simulink model "scenarioCloseLoop_supervisoryACC"  (R2019b)
settings: Solver=FixedStepAuto  StartTime=0.0  StopTime=30  FixedStep=0.01  RelTol=1e-3
PreLoadFcn:
  | Ts1 = 0.01;
  | Ts2 = 0.1;
InitFcn:
  | initACCParams_pid;
  | Ts1 = 0.01;
  | Ts2 = 0.1;
model workspace (MAT data in the model file):
  firstWarning = 1
  originalScenarioChecksum = '3C3E23DDE530CB8BEC76DD6DBB66960A'
undefined symbols (not defined in the file): APP_gain, BPP_gain, m, sigbuilder_block, steer_gain
libraries: drivingscenarioandsensors x2, autolibshared x1, vehdynlibviscommon x1
settings Model: SILPILSystemUnderTest=refmodels  EnablePacing=on  Creator=sseshadr  LastModifiedBy=cdsouza
settings OptimizationCC: DefaultParameterBehavior=Inlined  EnhancedBackFolding=on  PassReuseOutputArgsAs=Individual arguments  ZeroExternalMemoryAtStartup=off  ZeroInternalMemoryAtStartup=off  OptimizeBlockOrder=speed  DifferentSizesBufferReuse=on  OptimizationCustomize=off  EfficientTunableParamExpr=on
settings DebuggingCC: ParameterTunabilityLossMsg=error
settings SFSimCC: MATLABDynamicMemAlloc=off
settings RTWCC: SystemTargetFile=ert.tlc  TemplateMakefile=ert_default_tmf  GenerateReport=on  IncludeHyperlinkInReport=on  LaunchReport=on  PortableWordSizes=on  CreateSILPILBlock=SIL  CodeExecutionProfiling=on  CodeProfilingInstrumentation=coarse  GenerateTraceInfo=on  GenerateTraceReport=on  GenerateTraceReportSl=on  GenerateTraceReportSf=on  GenerateTraceReportEml=on
settings CodeAppCC: ForceParamTrailComments=on  IgnoreCustomStorageClasses=off  OperatorAnnotations=on  SimulinkDataObjDesc=on  SFDataObjDesc=on  InsertBlockDesc=on
settings ERTTargetCC: TargetLangStandard=C99 (ISO)  GenerateSampleERTMain=on  InlinedParameterPlacement=NonHierarchical  ERTCustomFileTemplate=example_file_process.tlc

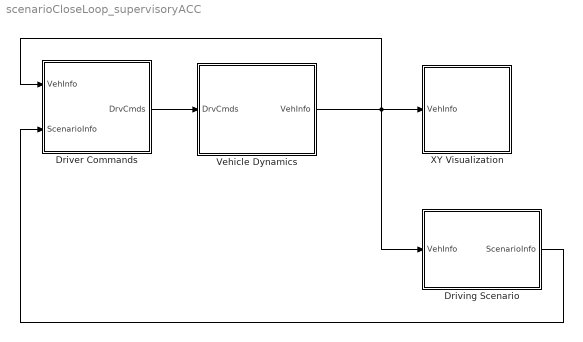
== system scenarioCloseLoop_supervisoryACC ==
  Driver Commands : Subsystem
  Driving Scenario : Subsystem
  Vehicle Dynamics : Subsystem
  XY Visualization : Subsystem
  wires:
  Driving Scenario/1(ScenarioInfo) -> Driver Commands/2(ScenarioInfo)
  Vehicle Dynamics/1(VehInfo) -> Driving Scenario/1(VehInfo), Driver Commands/1(VehInfo), XY Visualization/1(VehInfo)
  Driver Commands/1(DrvCmds) -> Vehicle Dynamics/1(DrvCmds)

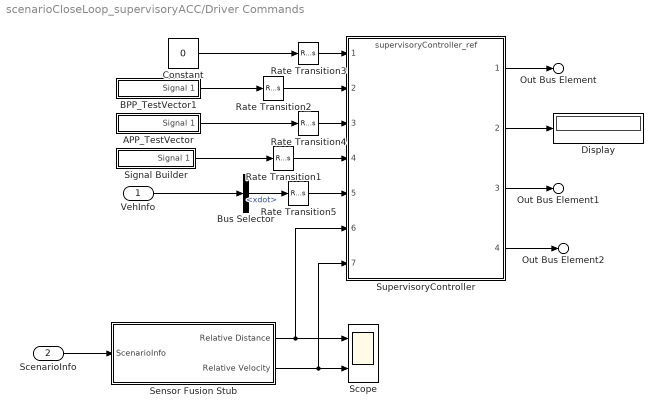
== system scenarioCloseLoop_supervisoryACC/Driver Commands ==
  VehInfo : Inport
  ScenarioInfo : Inport  Port=2
  APP_TestVector : Subsystem  Tag=STV Subsys  LoadFcn=sigbuilder_block('load');  StartFcn=sigbuilder_block('start');  StopFcn=sigbuilder_block('stop');  ClipboardFcn=sigbuilder_block('clipboard');  mask(Sigbuilder block){tuvar=[0:10]}
      mask help: Simulink:masks:SigbuilderBlock_MD
      mask init:
      | if ~strcmp(get_param(bdroot(gcbh),'SimulationStatus'),'stopped') tuvar = sigbuilder_block('maskInit'); end
      settings: CopyFcn=sigbuilder_block('copy');  DeleteFcn=sigbuilder_block('delete');  ModelCloseFcn=sigbuilder_block('modelClose');  PreSaveFcn=sigbuilder_block('preSave');  PauseFcn=sigbuilder_block('pause');  ContinueFcn=sigbuilder_block('continue');  NameChangeFcn=sigbuilder_block('namechange');  OpenFcn=sigbuilder_block('open',[609 515.25 550.5 237.75 ]);  CloseFcn=sigbuilder_block('close');
      mask Display: plot(0, 0, 100, 100,[2, 2, 32, 32, 2], [68, 8, 8, 68, 68],[32, 2], [38, 38], [32, 19, 2],[53, 60, 44], [32, 17, 17, 2],[16, 16, 31, 31]);txt = getActiveGroup(gcbh);text(2, 100, txt,'verticalAlignment', 'top');
  BPP_TestVector1 : Subsystem  Tag=STV Subsys  LoadFcn=sigbuilder_block('load');  StartFcn=sigbuilder_block('start');  StopFcn=sigbuilder_block('stop');  ClipboardFcn=sigbuilder_block('clipboard');  mask(Sigbuilder block){tuvar=[0:10]}
      mask help: Simulink:masks:SigbuilderBlock_MD
      mask init:
      | if ~strcmp(get_param(bdroot(gcbh),'SimulationStatus'),'stopped') tuvar = sigbuilder_block('maskInit'); end
      settings: CopyFcn=sigbuilder_block('copy');  DeleteFcn=sigbuilder_block('delete');  ModelCloseFcn=sigbuilder_block('modelClose');  PreSaveFcn=sigbuilder_block('preSave');  PauseFcn=sigbuilder_block('pause');  ContinueFcn=sigbuilder_block('continue');  NameChangeFcn=sigbuilder_block('namechange');  OpenFcn=sigbuilder_block('open',[325.5 304.5 550.5 278.25 ]);  CloseFcn=sigbuilder_block('close');
      mask Display: plot(0, 0, 100, 100,[2, 2, 32, 32, 2], [68, 8, 8, 68, 68],[32, 2], [38, 38], [32, 19, 2],[53, 60, 44], [32, 17, 17, 2],[16, 16, 31, 31]);txt = getActiveGroup(gcbh);text(2, 100, txt,'verticalAlignment', 'top');
  Bus Selector : BusSelector  OutputSignals=BdyFrm.Cg.Vel.xdot
  Constant : Constant  Value=0  SampleTime=0.01
  Display : Display
  Rate Transition{1..5} (5 alike) : RateTransition  OutPortSampleTime=0.01
  Scope : Scope  NumInputPorts=2
  Sensor Fusion Stub : Subsystem
  Signal Builder : Subsystem  Tag=STV Subsys  LoadFcn=sigbuilder_block('load');  StartFcn=sigbuilder_block('start');  StopFcn=sigbuilder_block('stop');  ClipboardFcn=sigbuilder_block('clipboard');  mask(Sigbuilder block){tuvar=[0:10]}
      mask help: Simulink:masks:SigbuilderBlock_MD
      mask init:
      | if ~strcmp(get_param(bdroot(gcbh),'SimulationStatus'),'stopped') tuvar = sigbuilder_block('maskInit'); end
      settings: CopyFcn=sigbuilder_block('copy');  DeleteFcn=sigbuilder_block('delete');  ModelCloseFcn=sigbuilder_block('modelClose');  PreSaveFcn=sigbuilder_block('preSave');  PauseFcn=sigbuilder_block('pause');  ContinueFcn=sigbuilder_block('continue');  NameChangeFcn=sigbuilder_block('namechange');  OpenFcn=sigbuilder_block('open',[401.25 280.5 550.5 278.25 ]);  CloseFcn=sigbuilder_block('close');
      mask Display: plot(0, 0, 100, 100,[2, 2, 32, 32, 2], [68, 8, 8, 68, 68],[32, 2], [38, 38], [32, 19, 2],[53, 60, 44], [32, 17, 17, 2],[16, 16, 31, 31]);txt = getActiveGroup(gcbh);text(2, 100, txt,'verticalAlignment', 'top');
  SupervisoryController : ModelReference  ModelNameDialog=supervisoryController_ref  SimulationMode=Normal  ModelReferenceVersion=1.30
  Out Bus Element : Outport  PortName=DrvCmds  Element=SteerCmd
  Out Bus Element1 : Outport  PortName=DrvCmds  Element=BPP Pedal
  Out Bus Element2 : Outport  PortName=DrvCmds  Element=APP Pedal
  wires:
  ScenarioInfo/1 -> Sensor Fusion Stub/1(ScenarioInfo)
  VehInfo/1 -> Bus Selector/1
  Sensor Fusion Stub/1(Relative Distance) -> SupervisoryController/6, Scope/1
  Sensor Fusion Stub/2(Relative Velocity) -> SupervisoryController/7, Scope/2
  Bus Selector/1 -> Rate Transition5/1  "<xdot>"
  SupervisoryController/1 -> Out Bus Element/1
  SupervisoryController/2 -> Display/1
  SupervisoryController/3 -> Out Bus Element1/1
  SupervisoryController/4 -> Out Bus Element2/1
  Rate Transition4/1 -> SupervisoryController/3
  Rate Transition2/1 -> SupervisoryController/2
  Rate Transition3/1 -> SupervisoryController/1
  Rate Transition5/1 -> SupervisoryController/5
  Signal Builder/1(Signal 1) -> Rate Transition1/1
  APP_TestVector/1(Signal 1) -> Rate Transition4/1
  Constant/1 -> Rate Transition3/1
  BPP_TestVector1/1(Signal 1) -> Rate Transition2/1
  Rate Transition1/1 -> SupervisoryController/4

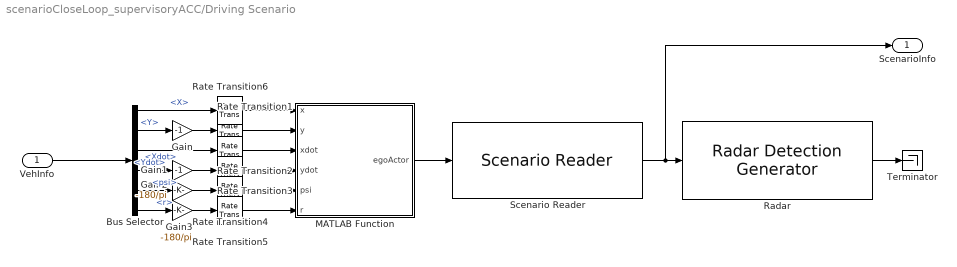
== system scenarioCloseLoop_supervisoryACC/Driving Scenario ==
  VehInfo : Inport
  Bus Selector : BusSelector  OutputSignals=InertFrm.Cg.Disp.X,InertFrm.Cg.Disp.Y,InertFrm.Cg.Vel.Xdot,InertFrm.Cg.Vel.Ydot,InertFrm.Cg.Ang.psi,BdyFrm.Cg.AngVel.r
  Gain : Gain  Gain=-1
  Gain1 : Gain  Gain=-1
  Gain2 : Gain  Gain=-180/pi
  Gain3 : Gain  Gain=-180/pi
  MATLAB Function : MATLAB Function  TreatAsAtomicUnit=on
  Radar : drivingscenarioandsensors/Radar Detection Generator  SensorIndex=1  UpdateInterval=0.1  SensorLocation=[3.5 0]  Height=0.2  Yaw=0  Pitch=0  Roll=0  BusNameSource=Auto  BusName=BusRadarDetectionGenerator  MaxNumDetectionsSource=Property  MaxNumDetections=50  DetectionCoordinates=Ego Cartesian  SimulateUsing=Interpreted execution  AzimuthResolution=4  ElevationResolution=10  RangeResolution=2.5  RangeRateResolution=0.5  AzimuthBiasFraction=0.1  ElevationBiasFraction=0.1  RangeBiasFraction=0.05  RangeRateBiasFraction=0.05  FieldOfView=[100 5]  MaxRange=50  RangeRateLimits=[-100 100]  DetectionProbability=0.9  FalseAlarmRate=1e-06  ReferenceRange=100  ReferenceRCS=0  HasElevation=off  HasRangeRate=on  HasNoise=on  HasFalseAlarms=on  HasOcclusion=on  InitialSeedSource=Repeatable  InitialSeed=0  UsedSeed=0  ActorProfilesSource=MATLAB expression  ActorProfilesParameters=driving.internal.ActorProfilesRadarParameters  ActorProfilesExpression=[struct('ActorID',1,'ClassID',1,'Length',4.7,'Width',1.8,'Height',1.4,'OriginOffset',[-1.35 0 0],'RCSPattern',[10 10;10 10],'RCSAzimuthAngles',[-180 180],'RCSElevationAngles',[-90 90]); struct('ActorID',2,'ClassID',1,'Length',4.7,'Width',1.8,'Height',1.4,'OriginOffset',[-1.35 0 0],'RCSPattern',[10 10;10 10],'RCSAzimuthAngles',[-180 180],'RCSElevationAngles',[-90 90]); struct('ActorID',3,'ClassID',1,'Length',4.7,'Width',1.8,'Height',1.4,'OriginOffset',[-1.35 0 0],'RCSPattern',[10 10;10 10],'RCSAzimuthAngles',[-180 180],'RCSElevationAngles',[-90 90]); struct('ActorID',4,'ClassID',1,'Length',4.7,'Width',1.8,'Height',1.4,'OriginOffset',[-1.35 0 0],'RCSPattern',[10 10;10 10],'RCSAzimuthAngles',[-180 180],'RCSElevationAngles',[-90 90])]
      settings: SourceProductName=Automated Driving Toolbox  SourceProductBaseCode=DR
  Rate Transition{1..6} (6 alike) : RateTransition  OutPortSampleTime=0.1
  Scenario Reader : drivingscenarioandsensors/Scenario Reader  ScenarioSource=From file  ScenarioFileName=Straight.mat  ScenarioVariableName=scenario  OutputCoordinateSystem=Vehicle coordinates  EgoVehicleSource=Input port  EgoVehicleActorID=1  SampleTime=0.1  LaneBoundaryOutput=None  LaneBoundaryDistance=0:0.5:9.5  LaneBoundaryLocation=Center of lane markings  BusNameSource=Auto  BusName=BusActors  BusName2Source=Auto  BusName2=BusLaneBoundaries  SimulateUsing=Interpreted execution
      settings: SourceProductName=Automated Driving Toolbox
  Terminator : Terminator
  ScenarioInfo : Outport
  wires:
  Bus Selector/3 -> Rate Transition2/1  "<Xdot>"
  Bus Selector/6 -> Gain3/1  "<r>"
  Bus Selector/1 -> Rate Transition6/1  "<X>"
  Bus Selector/2 -> Gain/1  "<Y>"
  Bus Selector/5 -> Gain2/1  "<psi>"
  VehInfo/1 -> Bus Selector/1
  Bus Selector/4 -> Gain1/1  "<Ydot>"
  Rate Transition6/1 -> MATLAB Function/1(x)
  Rate Transition1/1 -> MATLAB Function/2(y)
  Rate Transition2/1 -> MATLAB Function/3(xdot)
  Rate Transition3/1 -> MATLAB Function/4(ydot)
  Rate Transition4/1 -> MATLAB Function/5(psi)
  Rate Transition5/1 -> MATLAB Function/6(r)
  Radar/1 -> Terminator/1
  Scenario Reader/1 -> ScenarioInfo/1, Radar/1
  MATLAB Function/1(egoActor) -> Scenario Reader/1
  Gain/1 -> Rate Transition1/1
  Gain1/1 -> Rate Transition3/1
  Gain2/1 -> Rate Transition4/1
  Gain3/1 -> Rate Transition5/1

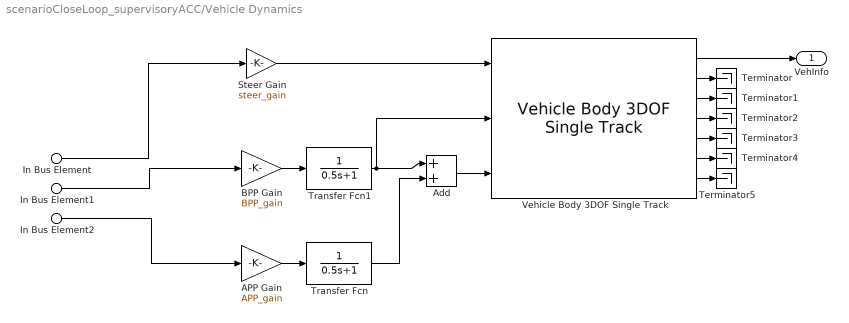
== system scenarioCloseLoop_supervisoryACC/Vehicle Dynamics ==
  In Bus Element : Inport  PortName=DrvCmds  Element=SteerCmd
  In Bus Element1 : Inport  PortName=DrvCmds  Element=BPP Pedal
  In Bus Element2 : Inport  PortName=DrvCmds  Element=APP Pedal
  APP Gain : Gain  Gain=APP_gain
  Add : Sum
  BPP Gain : Gain  Gain=BPP_gain
  Steer Gain : Gain  Gain=steer_gain
  Terminator{,1..5} (6 alike) : Terminator
  Transfer Fcn : TransferFcn  Denominator=[0.5 1]
  Transfer Fcn1 : TransferFcn  Denominator=[0.5 1]
  Vehicle Body 3DOF Single Track : autolibshared/Vehicle Body 3DOF Single Track  trackMode=Single (bicycle)  inputMode=External longitudinal forces  frontSteerMode=on  rearSteerMode=off  windMode=off  muMode=off  extFMode=off  extMMode=off  extXo=off  extpsio=off  extxdoto=off  extro=off  extYo=off  extTamb=off  extydoto=off  aMode=2  NF=2  NR=2  m=m  a=1.4  b=1.6  h=0.35  X_o=0  xdot_o=0  CalphaMode=off  sigmaMode=on  d=0  w=[1.4,1.4]  Cy_f=12e3  Cy_r=11e3  sigma_f=.1  sigma_r=.1  alpha_f_brk=[-.1 .1]  Cy_f_data=[-9e3 9e3]  alpha_r_brk=[-.1 .1]  Cy_r_data=[-9e3 9e3]  Y_o=0  ydot_o=0  Izz=4000  psi_o=0  r_o=0  Af=2  Cd=.3  Cl=.1  Cpm=.1  beta_w=[0:0.01:0.3]  Cs=[0:0.03:0.9]  Cym=[0:0.01:0.3]  Pabs=101325  Tair=273  g=9.81  mu=1  xdot_tol=.01  Fznom=5000  Fxtire_sat=7e4  Fytire_sat=7e4  longOff=0  latOff=0  vertOff=0  wrapAng=off
      settings: SourceProductName=Powertrain Blockset  SourceProductBaseCode=PW
  VehInfo : Outport
  wires:
  Vehicle Body 3DOF Single Track/7 -> Terminator5/1
  Transfer Fcn/1 -> Add/2
  Vehicle Body 3DOF Single Track/6 -> Terminator4/1
  BPP Gain/1 -> Transfer Fcn1/1
  In Bus Element1/1 -> BPP Gain/1
  Steer Gain/1 -> Vehicle Body 3DOF Single Track/1
  Vehicle Body 3DOF Single Track/4 -> Terminator2/1
  Vehicle Body 3DOF Single Track/2 -> Terminator/1
  Vehicle Body 3DOF Single Track/5 -> Terminator3/1
  Transfer Fcn1/1 -> Vehicle Body 3DOF Single Track/2, Add/1
  APP Gain/1 -> Transfer Fcn/1
  Vehicle Body 3DOF Single Track/3 -> Terminator1/1
  Add/1 -> Vehicle Body 3DOF Single Track/3
  Vehicle Body 3DOF Single Track/1 -> VehInfo/1
  In Bus Element/1 -> Steer Gain/1
  In Bus Element2/1 -> APP Gain/1

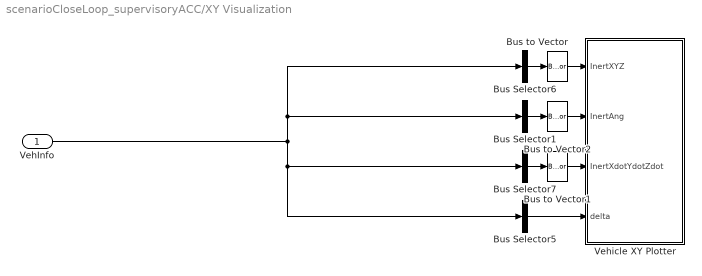
== system scenarioCloseLoop_supervisoryACC/XY Visualization ==
  VehInfo : Inport
  Bus Selector1 : BusSelector  OutputSignals=InertFrm.Cg.Ang.phi,InertFrm.Cg.Ang.theta,InertFrm.Cg.Ang.psi  OutputAsBus=on
  Bus Selector5 : BusSelector  OutputSignals=BdyFrm.FrntAxl.Steer.WhlAngFL,BdyFrm.FrntAxl.Steer.WhlAngFR,BdyFrm.RearAxl.Steer.WhlAngRL,BdyFrm.RearAxl.Steer.WhlAngRR  OutputAsBus=on
  Bus Selector6 : BusSelector  OutputSignals=InertFrm.Geom.Disp.X,InertFrm.Geom.Disp.Y,InertFrm.Geom.Disp.Z  OutputAsBus=on
  Bus Selector7 : BusSelector  OutputSignals=InertFrm.Geom.Vel.Xdot,InertFrm.Geom.Vel.Ydot,InertFrm.Geom.Vel.Zdot  OutputAsBus=on
  Bus to Vector : BusToVector
  Bus to Vector1 : BusToVector
  Bus to Vector2 : BusToVector
  Vehicle XY Plotter : Subsystem  mask(Vehicle XY Plotter){a=2, b=2, w=2, figBorder=10, bufferSize=1024, extRef=off, pltDT=.1}
      mask prompts: a "Distance to front axle from CG, a [m]:"; b "Distance to rear axle from CG, b [m]:"; w "Track width, w [m]:"; figBorder "Distance to figure borders, figBorder [m]:"; bufferSize "Path buffer sampe size, bufferSize []:"; extRef "Plot path reference, extRef"; pltDT "Plot update rate, pltDT [s]:"
      mask help:
      | This block will display a MATLAB figure which indicates the vehicle path, current position and heading velocity.
      | An optional path reference is also provided.
      mask init:
      | if autoblkschecksimstopped(gcb)
      |     PortName = 'RefXYZ';
      |     InportOption  = {'built-in/Ground', [PortName, ' Ground'];...
      |         'built-in/Inport',PortName };
      |     if ~strcmp(get_param(gcb,'extRef'),'on')
      |         NewBlkHdl = autoblksreplaceblock(gcb, InportOption, 1);
      |         set_param(NewBlkHdl, 'ShowName', 'off');
      |     else
      |         autoblksreplaceblock(gcb, InportOption, 2);
      |     end
      | end
      mask TypeOptions a: Vehicle XY Plotter/a
      mask TypeOptions b: Vehicle XY Plotter/b
      mask TypeOptions w: Vehicle XY Plotter/w
      mask TypeOptions figBorder: Vehicle XY Plotter/figBorder
      mask TypeOptions bufferSize: Vehicle XY Plotter/bufferSize
  wires:
  Bus Selector5/1 -> Vehicle XY Plotter/4(delta)
  Bus Selector7/1 -> Bus to Vector1/1
  Bus Selector6/1 -> Bus to Vector/1
  Bus to Vector2/1 -> Vehicle XY Plotter/2(InertAng)
  Bus Selector1/1 -> Bus to Vector2/1
  Bus to Vector/1 -> Vehicle XY Plotter/1(InertXYZ)
  Bus to Vector1/1 -> Vehicle XY Plotter/3(InertXdotYdotZdot)
  VehInfo/1 -> Bus Selector5/1, Bus Selector7/1, Bus Selector6/1, Bus Selector1/1

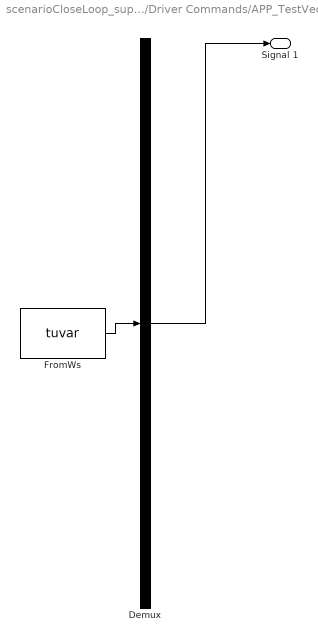
== system scenarioCloseLoop_supervisoryACC/Driver Commands/APP_TestVector ==
  Demux : Demux  Tag=STV Demux  Outputs=1
  FromWs : FromWorkspace  Tag=STV FromWs  VariableName=tuvar  SampleTime=0
      SigBuilderData=|
      | common.afterFinalStr = 'Extrapolate'
      | common.sampleTime = 0
      | dataSet.timeRange = [0 10]
      | dataSet.name = 'Group 1'
      | sbobj.Groups.Name = 'Group 1'
      | sbobj.Groups.Signals.Name = 'Signal 1'
      | sbobj.Groups.Signals.XData = [0 1 2 2.2 4 6 10]
      | sbobj.Groups.Signals.YData = [0.8 0.19 0.6 0 0 0 0]
  Signal 1 : Outport  Tag=STV Outport
  wires:
  FromWs/1 -> Demux/1
  Demux/1 -> Signal 1/1

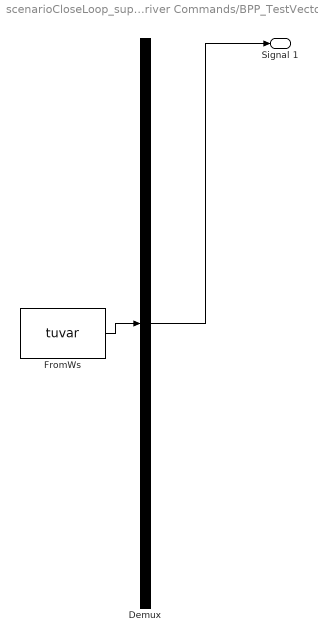
== system scenarioCloseLoop_supervisoryACC/Driver Commands/BPP_TestVector1 ==
  Demux : Demux  Tag=STV Demux  Outputs=1
  FromWs : FromWorkspace  Tag=STV FromWs  VariableName=tuvar  SampleTime=0
      SigBuilderData=|
      | common.afterFinalStr = 'Extrapolate'
      | common.sampleTime = 0
      | dataSet.timeRange = [0 10]
      | dataSet.name = 'Group 1'
      | sbobj.Groups.Name = 'Group 1'
      | sbobj.Groups.Signals.Name = 'Signal 1'
      | sbobj.Groups.Signals.XData = [0 1 2 2.2 4 6 10]
      | sbobj.Groups.Signals.YData = [0 0.4 0 0 0 0 0]
  Signal 1 : Outport  Tag=STV Outport
  wires:
  Demux/1 -> Signal 1/1
  FromWs/1 -> Demux/1

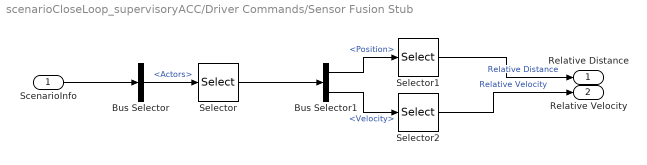
== system scenarioCloseLoop_supervisoryACC/Driver Commands/Sensor Fusion Stub ==
  ScenarioInfo : Inport
  Bus Selector : BusSelector  OutputSignals=Actors
  Bus Selector1 : BusSelector  OutputSignals=Position,Velocity
  Selector : Selector  InputPortWidth=3  IndexOptions=Index vector (dialog)  Indices=3  OutputSizes=1
  Selector1 : Selector  InputPortWidth=3  IndexOptions=Index vector (dialog)  Indices=1  OutputSizes=1
  Selector2 : Selector  InputPortWidth=3  IndexOptions=Index vector (dialog)  Indices=1  OutputSizes=1
  Relative Distance : Outport
  Relative Velocity : Outport  Port=2
  wires:
  Selector/1 -> Bus Selector1/1
  Selector2/1 -> Relative Velocity/1  "Relative Velocity"
  ScenarioInfo/1 -> Bus Selector/1
  Bus Selector/1 -> Selector/1  "<Actors>"
  Selector1/1 -> Relative Distance/1  "Relative Distance"
  Bus Selector1/1 -> Selector1/1  "<Position>"
  Bus Selector1/2 -> Selector2/1  "<Velocity>"

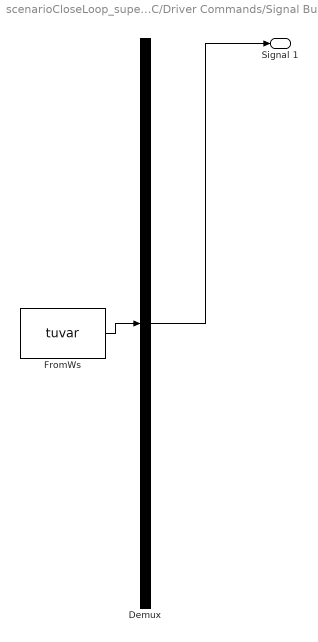
== system scenarioCloseLoop_supervisoryACC/Driver Commands/Signal Builder ==
  Demux : Demux  Tag=STV Demux  Outputs=1
  FromWs : FromWorkspace  Tag=STV FromWs  VariableName=tuvar  SampleTime=0
      SigBuilderData=|
      | common.afterFinalStr = 'Extrapolate'
      | common.sampleTime = 0
      | dataSet.timeRange = [0 10]
      | dataSet.name = 'Group 1'
      | sbobj.Groups.Name = 'Group 1'
      | sbobj.Groups.Signals.Name = 'Signal 1'
      | sbobj.Groups.Signals.XData = [0 2.15 2.15 2.2 2.2 4 6 6 10]
      | sbobj.Groups.Signals.YData = [-1 -1 180 180 -1 -1 1 0 0]
  Signal 1 : Outport  Tag=STV Outport
  wires:
  Demux/1 -> Signal 1/1
  FromWs/1 -> Demux/1

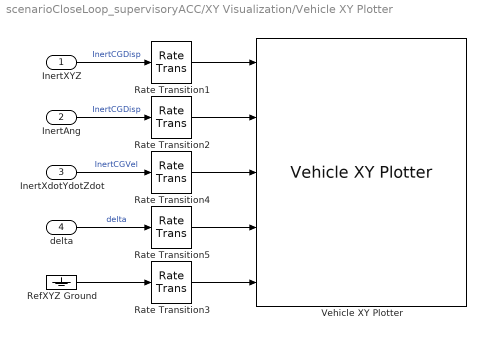
== system scenarioCloseLoop_supervisoryACC/XY Visualization/Vehicle XY Plotter ==
  InertXYZ : Inport
  InertAng : Inport  Port=2
  InertXdotYdotZdot : Inport  Port=3
  delta : Inport  Port=4
  Rate Transition{1..5} (5 alike) : RateTransition  Deterministic=off  OutPortSampleTime=pltDT
  RefXYZ Ground : Ground
  Vehicle XY Plotter : vehdynlibviscommon/Vehicle XY Plotter  bufferSize=bufferSize  w=w  a=a  b=b  figBorder=figBorder
      settings: SourceProductName=Vehicle Dynamics Blockset  SourceProductBaseCode=VE
  wires:
  Rate Transition5/1 -> Vehicle XY Plotter/4
  Rate Transition4/1 -> Vehicle XY Plotter/3
  Rate Transition2/1 -> Vehicle XY Plotter/2
  Rate Transition1/1 -> Vehicle XY Plotter/1
  Rate Transition3/1 -> Vehicle XY Plotter/5
  delta/1 -> Rate Transition5/1  "delta"
  InertXYZ/1 -> Rate Transition1/1  "InertCGDisp"
  InertXdotYdotZdot/1 -> Rate Transition4/1  "InertCGVel"
  InertAng/1 -> Rate Transition2/1  "InertCGDisp"
  RefXYZ Ground/1 -> Rate Transition3/1

== matlab function scenarioCloseLoop_supervisoryACC/Driving Scenario/MATLAB Function ==
  data: x input; egoActor output Bus: BusActors1Actors; y input; xdot input; ydot input; psi input; r input
function egoActor = packActor(x,y,xdot,ydot,psi,r)

egoActor = struct(...
    'ActorID',1,...
    'Position', [x y 0], ...
    'Velocity', [xdot ydot 0], ...
    'Roll', 0, ...
    'Pitch', 0, ...
    'Yaw', psi, ...
    'AngularVelocity', [0 0 r]);
